simulink model "SMCmodel"  (R2020b)
settings: Solver=VariableStepAuto  StartTime=0.0  StopTime=10.0  FixedStep=0.00005  MaxStep=0.02  MinStep=0.00001  RelTol=1e-3  EnableMultiTasking=on
undefined symbols (not defined in the file): a, B, beta, cond_init, d, delta, g, J, Ke, Kt, L, m, Ra
libraries: simulink x1
settings Model: Creator=Administrador  LastModifiedBy=andre
settings DataIOCC: LimitDataPoints=on  SaveFormat=Array  SignalLoggingSaveFormat=ModelDataLogs  ReturnWorkspaceOutputs=off
settings OptimizationCC: ExpressionDepthLimit=2147483647  InitFltsAndDblsToZero=on  LifeSpan=inf
settings DebuggingCC: UnderspecifiedInitializationDetection=Classic  MergeDetectMultiDrivingBlocksExec=none  SolverPrmCheckMsg=warning  FcnCallInpInsideContextMsg=warning  StateNameClashWarn=warning  SFUnexpectedBacktrackingDiag=warning  SFNoUnconditionalDefaultTransitionDiag=warning  SFExecutionAtInitializationDiag=none  ArithmeticOperatorsInVariantConditions=warning
settings HardwareCC: ProdBitPerPointer=32  ProdBitPerSizeT=32  ProdBitPerPtrDiffT=32  ProdLargestAtomicFloat=None  ProdIntDivRoundTo=Undefined  ProdEndianess=Unspecified  ProdWordSize=32  ProdHWDeviceType=32-bit Generic
settings ModelReferenceCC: PropagateSignalLabelsOutOfModel=off
settings SFSimCC: SimUseLocalCustomCode=off  CustomCodeUndefinedFunction=UseInterfaceOnly
settings RTWCC: RTWUseLocalCustomCode=off
settings CodeAppCC: StateflowObjectComments=on
settings GRTTargetCC: TargetLangStandard=C89/C90 (ANSI)  CombineOutputUpdateFcns=off  GRTInterface=on
settings ConfigComp: CovMetricSettings=dw  CovSaveCumulativeToWorkspaceVar=on  CovSaveSingleToWorkspaceVar=on  CovExternalEMLEnable=off

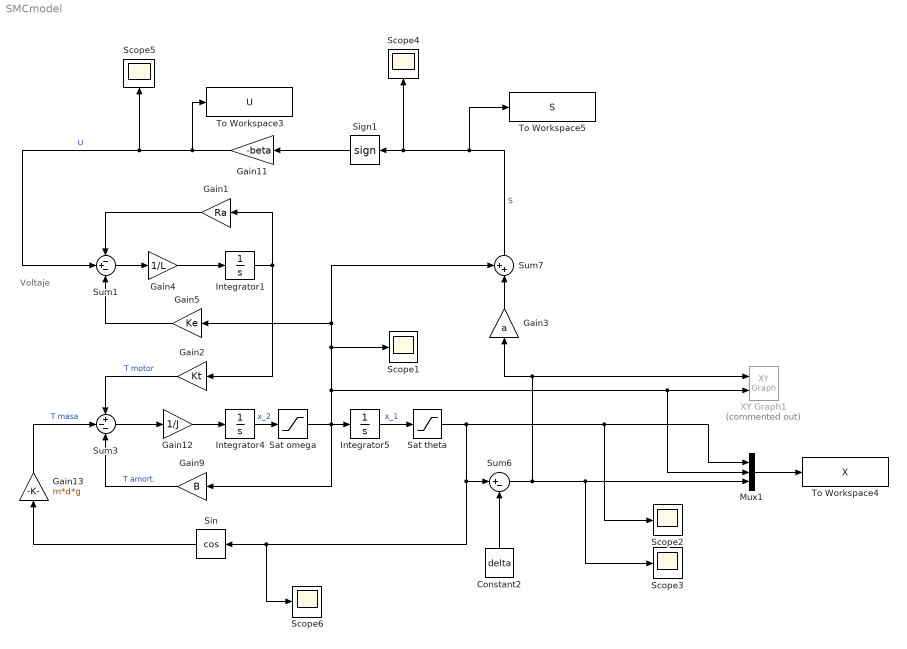
== system SMCmodel ==
  note: Voltaje
  Constant2 : Constant  Value=delta
  Gain1 : Gain  Gain=Ra
  Gain11 : Gain  Gain=-beta
  Gain12 : Gain  Gain=1/J
  Gain13 : Gain  Gain=m*d*g
  Gain2 : Gain  Gain=Kt
  Gain3 : Gain  Gain=a
  Gain4 : Gain  Gain=1/L
  Gain5 : Gain  Gain=Ke
  Gain9 : Gain  Gain=B
  Integrator1 : Integrator
  Integrator4 : Integrator
  Integrator5 : Integrator  InitialCondition=cond_init
  Mux1 : Mux  Inputs=3
  Sat omega : Saturate  UpperLimit=pi/2  LowerLimit=-pi/2
  Sat theta : Saturate  UpperLimit=pi  LowerLimit=-pi
  Scope{1..6} (6 alike) : Scope
  Sign1 : Signum  ZeroCross=off
  Sin : Trigonometry  Operator=cos
  Sum1 : Sum  Inputs=-+-
  Sum3 : Sum  Inputs=+--
  Sum6 : Sum  Inputs=|+-
  Sum7 : Sum  Inputs=++|
  To Workspace3 : ToWorkspace  VariableName=U  SaveFormat=Timeseries  SampleTime=-1
  To Workspace4 : ToWorkspace  VariableName=X  SaveFormat=Timeseries  SampleTime=-1
  To Workspace5 : ToWorkspace  VariableName=S  SaveFormat=Timeseries  SampleTime=-1
  XY Graph1 : simulink/Sinks/XY Graph  Commented=on  xmin=-3  xmax=1  ymin=-1  ymax=5  st=-1
  wires:
  Constant2/1 -> Sum6/2
  Sign1/1 -> Gain11/1
  Gain13/1 -> Sum3/2  "T masa"
  Gain9/1 -> Sum3/3  "T amort."
  Integrator1/1 -> Gain2/1, Gain1/1
  Gain12/1 -> Integrator4/1
  Gain4/1 -> Integrator1/1
  Sin/1 -> Gain13/1
  Sum1/1 -> Gain4/1
  Sum3/1 -> Gain12/1
  Gain5/1 -> Sum1/3
  Integrator4/1 -> Sat omega/1  "x_2"
  Gain2/1 -> Sum3/1  "T motor"
  Gain1/1 -> Sum1/1
  Gain11/1 -> To Workspace3/1, Scope5/1, Sum1/2  "U"
  Integrator5/1 -> Sat theta/1  "x_1"
  Mux1/1 -> To Workspace4/1
  Sum7/1 -> To Workspace5/1, Scope4/1, Sign1/1  "S"
  Gain3/1 -> Sum7/2
  Sum6/1 -> Gain3/1, XY Graph1/1, Scope3/1, Mux1/3
  Sat omega/1 -> Mux1/2, XY Graph1/2, Scope1/1, Gain5/1, Sum7/1, Integrator5/1, Gain9/1
  Sat theta/1 -> Scope6/1, Sin/1, Sum6/1, Scope2/1, Mux1/1
